simulink model "Wiper_System_stateflow"  (R2022b)
settings: Solver=FixedStepDiscrete  StartTime=0.0  StopTime=10.0  FixedStep=0.1  RelTol=1e-3
model workspace (MAT data in the model file):
  Param = Simulink.Parameter
  Param.Value = 0.4
  Param.DataType = 'auto'
  Param.Complexity = 'real'
  Param.Dimensions = [1 1]
  WprSys_WprMotDutCycHighSpd = 0.7
  WprSys_WprMotDutCycHighSpd_SC = 0.7
  WprSys_WprMotDutCycLowSpd = 0.4
  WprSys_WprMotDutCycLowSpd_SC = 0.4
  WprSys_deltaSatVal = 0.05
  WprSys_vWprSnsrErrRead_SC = Simulink.Parameter
  WprSys_vWprSnsrErrRead_SC.Value = [0 0.1 0.2 0.3 0.4 0.5 0.6 0.7 0.7 0.7 0.7]
  WprSys_vWprSnsrErrRead_SC.DataType = 'single'
  WprSys_vWprSnsrErrRead_SC.Complexity = 'real'
  WprSys_vWprSnsrErrRead_SC.Dimensions = [1 11]
  WprSys_vWprSpdRqust_SC = Simulink.Parameter
  WprSys_vWprSpdRqust_SC.Value = [0; 0.1; 0.2; 0.3; 0.4; 0.5; 0.6; 0.7; 0.8; 0.9; 1]
  WprSys_vWprSpdRqust_SC.DataType = 'single'
  WprSys_vWprSpdRqust_SC.Complexity = 'real'
  WprSys_vWprSpdRqust_SC.Dimensions = [11 1]
undefined symbols (not defined in the file): Counter_timer, Stateflow_Counter
settings Model: Creator=Mohamed Wahdan  LastModifiedBy=Mohamed Wahdan

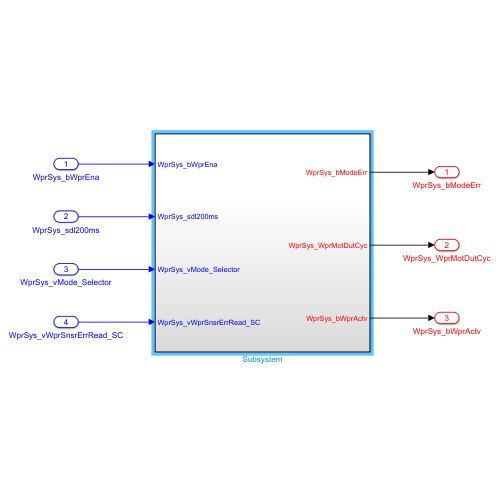
[thumbnail: Simulink's stored preview of the top-level diagram]
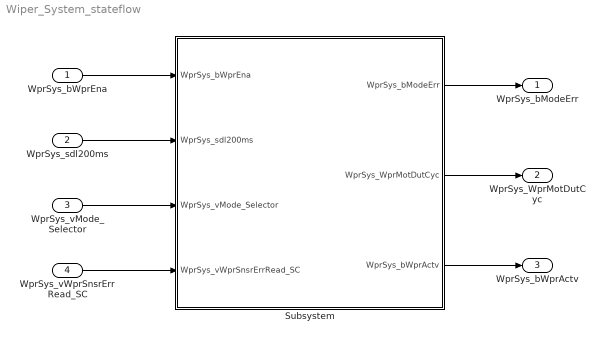
== system Wiper_System_stateflow ==
  WprSys_bWprEna : Inport
  WprSys_sdl200ms : Inport  Port=2
  WprSys_vMode_Selector : Inport  Port=3
  WprSys_vWprSnsrErrRead_SC : Inport  Port=4
  Subsystem : Subsystem
  WprSys_bModeErr : Outport
  WprSys_WprMotDutCyc : Outport  Port=2
  WprSys_bWprActv : Outport  Port=3
  wires:
  WprSys_bWprEna/1 -> Subsystem/1(WprSys_bWprEna)
  WprSys_sdl200ms/1 -> Subsystem/2(WprSys_sdl200ms)
  WprSys_vMode_Selector/1 -> Subsystem/3(WprSys_vMode_Selector)
  WprSys_vWprSnsrErrRead_SC/1 -> Subsystem/4(WprSys_vWprSnsrErrRead_SC)
  Subsystem/1(WprSys_bModeErr) -> WprSys_bModeErr/1
  Subsystem/2(WprSys_WprMotDutCyc) -> WprSys_WprMotDutCyc/1
  Subsystem/3(WprSys_bWprActv) -> WprSys_bWprActv/1

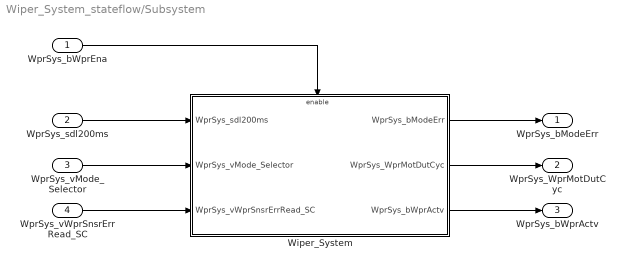
== system Wiper_System_stateflow/Subsystem ==
  WprSys_bWprEna : Inport
  WprSys_sdl200ms : Inport  Port=2
  WprSys_vMode_Selector : Inport  Port=3
  WprSys_vWprSnsrErrRead_SC : Inport  Port=4
  Wiper_System : Subsystem
  WprSys_bModeErr : Outport
  WprSys_WprMotDutCyc : Outport  Port=2
  WprSys_bWprActv : Outport  Port=3
  wires:
  Wiper_System/1(WprSys_bModeErr) -> WprSys_bModeErr/1
  WprSys_vMode_Selector/1 -> Wiper_System/2(WprSys_vMode_Selector)
  WprSys_bWprEna/1 -> Wiper_System/Enable
  Wiper_System/3(WprSys_bWprActv) -> WprSys_bWprActv/1
  Wiper_System/2(WprSys_WprMotDutCyc) -> WprSys_WprMotDutCyc/1
  WprSys_vWprSnsrErrRead_SC/1 -> Wiper_System/3(WprSys_vWprSnsrErrRead_SC)
  WprSys_sdl200ms/1 -> Wiper_System/1(WprSys_sdl200ms)

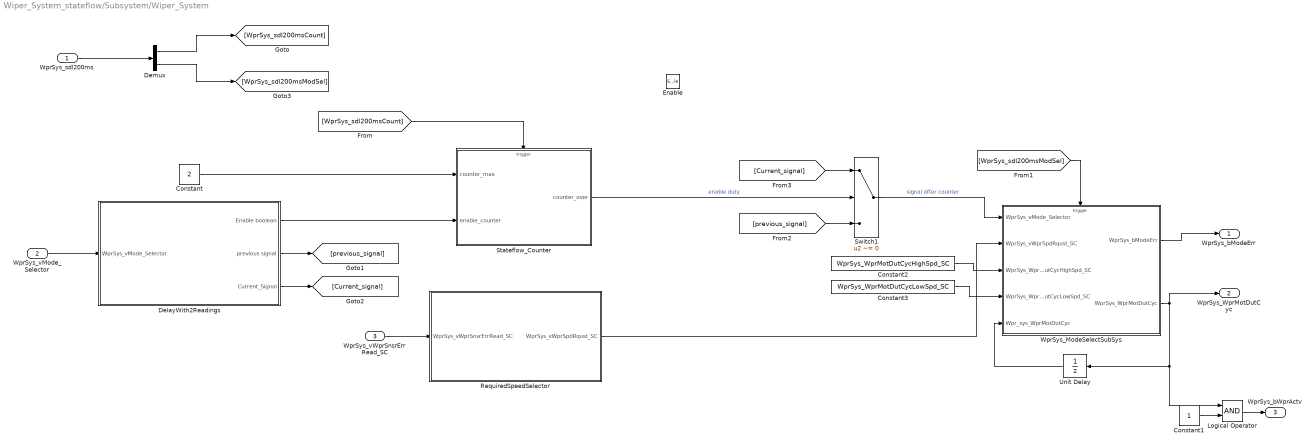
== system Wiper_System_stateflow/Subsystem/Wiper_System ==
  WprSys_sdl200ms : Inport
  WprSys_vMode_Selector : Inport  Port=2
  WprSys_vWprSnsrErrRead_SC : Inport  Port=3
  Enable : EnablePort
  Constant : Constant  Value=2
  Constant1 : Constant
  Constant2 : Constant  Value=WprSys_WprMotDutCycHighSpd_SC
  Constant3 : Constant  Value=WprSys_WprMotDutCycLowSpd_SC
  DelayWith2Readings : Subsystem
  Demux : Demux  Outputs=2
  Logical Operator : Logic  AllPortsSameDT=off  OutDataTypeStr=boolean
  RequiredSpeedSelector : Subsystem
  Stateflow_Counter : Stateflow chart  AncestorBlock=Counter_timer/Stateflow_Counter  TreatAsAtomicUnit=on
      settings: LibrarySourceBlock=Counter_timer/Stateflow_Counter
  Switch1 : Switch  Criteria=u2 ~= 0  SaturateOnIntegerOverflow=off  InputSameDT=off
  Unit Delay : UnitDelay  SampleTime=-1  HasFrameUpgradeWarning=on
  WprSys_ModeSelectSubSys : Stateflow chart  TreatAsAtomicUnit=on
  WprSys_bModeErr : Outport
  WprSys_WprMotDutCyc : Outport  Port=2
  WprSys_bWprActv : Outport  Port=3
  wires:
  [WprSys_sdl200msCount] -> Stateflow_Counter/Trigger
  WprSys_ModeSelectSubSys/2(WprSys_WprMotDutCyc) -> Logical Operator/1, Unit Delay/1, WprSys_WprMotDutCyc/1
  WprSys_sdl200ms/1 -> Demux/1
  [WprSys_sdl200msModSel] -> WprSys_ModeSelectSubSys/Trigger
  WprSys_ModeSelectSubSys/1(WprSys_bModeErr) -> WprSys_bModeErr/1
  Constant/1 -> Stateflow_Counter/1(counter_max)
  Stateflow_Counter/1(counter_over) -> Switch1/2  "enable duty"
  DelayWith2Readings/1(Enable boolean) -> Stateflow_Counter/2(enable_counter)
  Switch1/1 -> WprSys_ModeSelectSubSys/1(WprSys_vMode_Selector)  "signal after counter"
  DelayWith2Readings/2(previous signal) -> [previous_signal]
  [Current_signal] -> Switch1/1
  DelayWith2Readings/3(Current_Signal) -> [Current_signal]
  [previous_signal] -> Switch1/3
  WprSys_vMode_Selector/1 -> DelayWith2Readings/1(WprSys_vMode_Selector)
  Unit Delay/1 -> WprSys_ModeSelectSubSys/5(Wpr_sys_WprMotDutCyc)
  WprSys_vWprSnsrErrRead_SC/1 -> RequiredSpeedSelector/1(WprSys_vWprSnsrErrRead_SC)
  RequiredSpeedSelector/1(WprSys_vWprSpdRqust_SC) -> WprSys_ModeSelectSubSys/2(WprSys_vWprSpdRqust_SC)
  Constant1/1 -> Logical Operator/2
  Logical Operator/1 -> WprSys_bWprActv/1
  Demux/1 -> [WprSys_sdl200msCount]
  Demux/2 -> [WprSys_sdl200msModSel]
  Constant2/1 -> WprSys_ModeSelectSubSys/3(WprSys_WprMotDutCycHighSpd_SC)
  Constant3/1 -> WprSys_ModeSelectSubSys/4(WprSys_WprMotDutCycLowSpd_SC)

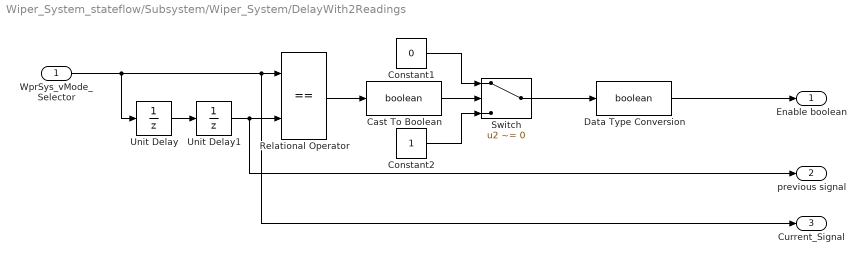
== system Wiper_System_stateflow/Subsystem/Wiper_System/DelayWith2Readings ==
  WprSys_vMode_Selector : Inport
  Cast To Boolean : DataTypeConversion  OutDataTypeStr=boolean  SaturateOnIntegerOverflow=off  RndMeth=Floor
  Constant1 : Constant  Value=0
  Constant2 : Constant
  Data Type Conversion : DataTypeConversion  OutDataTypeStr=boolean  SaturateOnIntegerOverflow=off  RndMeth=Floor
  Relational Operator : RelationalOperator  Operator===  OutDataTypeStr=boolean  RndMeth=Simplest  InputSameDT=off
  Switch : Switch  Criteria=u2 ~= 0  SaturateOnIntegerOverflow=off  InputSameDT=off
  Unit Delay : UnitDelay  SampleTime=-1  HasFrameUpgradeWarning=on
  Unit Delay1 : UnitDelay  SampleTime=-1  HasFrameUpgradeWarning=on
  Enable boolean : Outport
  previous signal : Outport  Port=2
  Current_Signal : Outport  Port=3
  wires:
  Constant2/1 -> Switch/3
  Unit Delay/1 -> Unit Delay1/1
  Unit Delay1/1 -> previous signal/1, Relational Operator/2
  Cast To Boolean/1 -> Switch/2
  Constant1/1 -> Switch/1
  Switch/1 -> Data Type Conversion/1
  Relational Operator/1 -> Cast To Boolean/1
  Data Type Conversion/1 -> Enable boolean/1
  WprSys_vMode_Selector/1 -> Unit Delay/1, Current_Signal/1, Relational Operator/1

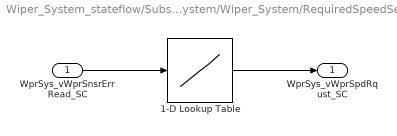
== system Wiper_System_stateflow/Subsystem/Wiper_System/RequiredSpeedSelector ==
  WprSys_vWprSnsrErrRead_SC : Inport
  1-D Lookup Table : Lookup_n-D  NumberOfTableDimensions=1  BreakpointsForDimension1=WprSys_vWprSpdRqust_SC  Table=WprSys_vWprSnsrErrRead_SC  InterpMethod=Linear Lagrange  InternalRulePriority=Speed  RndMeth=Simplest
  WprSys_vWprSpdRqust_SC : Outport
  wires:
  1-D Lookup Table/1 -> WprSys_vWprSpdRqust_SC/1
  WprSys_vWprSnsrErrRead_SC/1 -> 1-D Lookup Table/1

== stateflow chart Wiper_System_stateflow/Subsystem/Wiper_System/Stateflow_Counter ==
  settings: executeAtInitialization=1
  state Counter_on
    counter_over=false;
    counter = counter+1;
  state counter_reset
    counter=0;
  (default) -> counter_reset : {counter=0;}
  Counter_on -> counter_reset [order 1] : [counter==counter_max]{counter_over=true;}
  counter_reset -> Counter_on [order 1] : [enable_counter==1]
  Counter_on -> counter_reset [order 2] : [enable_counter==0]
  counter_reset -> (junction 33) [order 2]
  data: counter_max input; counter_over output boolean; enable_counter input boolean; counter local
  events: trigger200ms input EITHER_EDGE_EVENT

== stateflow chart Wiper_System_stateflow/Subsystem/Wiper_System/WprSys_ModeSelectSubSys ==
  settings: executeAtInitialization=1
  state Wiper
    state Off_Mode
      WprSys_WprMotDutCyc=0;
    state Auto_Mode
      state Below_sat
        WprSys_WprMotDutCyc=WprSys_WprMotDutCyc+delta;
      state Above_sat
        WprSys_WprMotDutCyc=WprSys_WprMotDutCyc+delta;
      state Within_Sat
        WprSys_WprMotDutCyc=WprSys_WprMotDutCyc+delta;
      (junction 53) -> Below_sat [order 1] : [delta<=-WprSys_deltaSatVal]{delta=-WprSys_deltaSatVal}
      (default) -> (junction 53)
      Auto_Mode -> (junction 53)
      (junction 53) -> Above_sat [order 2] : [delta>=WprSys_deltaSatVal]{delta=WprSys_deltaSatVal}
      (junction 53) -> Within_Sat [order 3]
    state Error_Mode
      WprSys_bModeErr=true;
    state High_Speed
      WprSys_WprMotDutCyc=WprSys_WprMotDutCycHighSpd_SC;
    state Low_Speed
      WprSys_WprMotDutCyc=WprSys_WprMotDutCycLowSpd_SC;
    Wiper -> (junction 7)
    (junction 7) -> Off_Mode [order 1] : [WprSys_vMode_Selector==0]
    (junction 7) -> Error_Mode [order 5]
    (default) -> (junction 7) : {WprSys_bModeErr=false;}
    (junction 7) -> Low_Speed [order 2] : [WprSys_vMode_Selector==1]
    (junction 7) -> High_Speed [order 3] : [WprSys_vMode_Selector==2]
    (junction 7) -> Auto_Mode [order 4] : [WprSys_vMode_Selector==3]{delta=WprSys_vWprSpdRqust_SC-Wpr_sys_WprMotDutCyc;}
  data: WprSys_vMode_Selector input; WprSys_vWprSpdRqust_SC input; WprSys_bModeErr output boolean; WprSys_WprMotDutCyc output; delta local; WprSys_deltaSatVal local double; WprSys_WprMotDutCycHighSpd_SC input; data local; WprSys_WprMotDutCycLowSpd_SC input; Wpr_sys_WprMotDutCyc input
  events: trigger200ms input EITHER_EDGE_EVENT
